simulink model "Bands6"  (R2018a)
settings: Solver=VariableStepAuto  StartTime=0.0  StopTime=0.01  RelTol=1e-3
undefined symbols (not defined in the file): fdesignblkfcn, G1, G2, G3, G4, G5, G6, gcbh, get, T
libraries: dspsrcs4 x1, dspxfrm3 x1, dspobslib x1
(part 1 of 2)
settings Model: Creator=Daniel  LastModifiedBy=Daniel

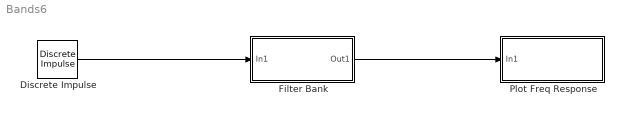
== system Bands6 ==
  Discrete Impulse : dspsrcs4/Discrete  Impulse  Delay=0  SampleTime=T  FrameSample=128  OutputFrames=off  dataType=double  isSigned=on  wordLen=16  udDataType=sfix(16)  fracBitsMode=Best precision  numFracBits=15  OutDataTypeStr=double  LastOutDataTypeStr=double
  "Filter Bank " : Subsystem
  Plot Freq Response : Subsystem
  wires:
  Discrete Impulse/1 -> "Filter Bank "/1(In1)
  "Filter Bank "/1(Out1) -> Plot Freq Response/1(In1)

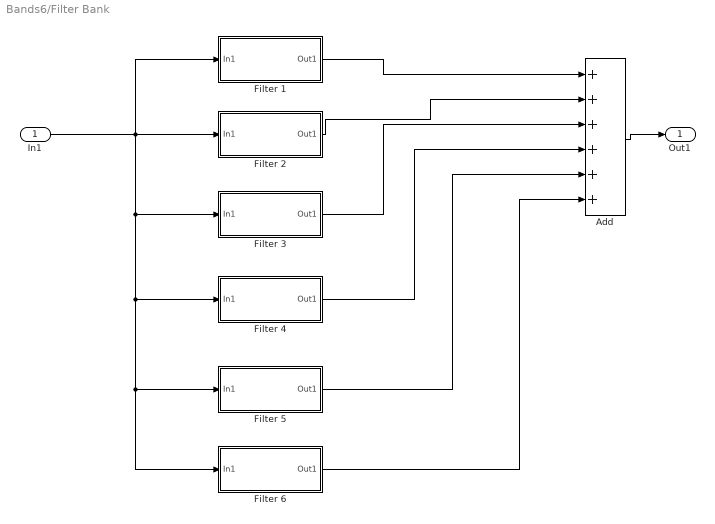
== system Bands6/Filter Bank  ==
  In1 : Inport
  Add : Sum  Inputs=++++++
  Filter 1 : Subsystem
  Filter 2 : Subsystem
  Filter 3 : Subsystem
  Filter 4 : Subsystem
  Filter 5 : Subsystem
  Filter 6 : Subsystem
  Out1 : Outport
  wires:
  In1/1 -> Filter 3/1(In1), Filter 6/1(In1), Filter 5/1(In1), Filter 4/1(In1), Filter 1/1(In1), Filter 2/1(In1)
  Add/1 -> Out1/1
  Filter 1/1(Out1) -> Add/1
  Filter 2/1(Out1) -> Add/2
  Filter 3/1(Out1) -> Add/3
  Filter 4/1(Out1) -> Add/4
  Filter 5/1(Out1) -> Add/5
  Filter 6/1(Out1) -> Add/6

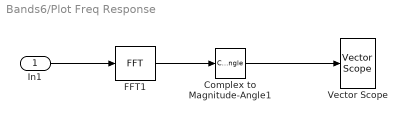
== system Bands6/Plot Freq Response ==
  In1 : Inport
  Complex to Magnitude-Angle1 : ComplexToMagnitudeAngle  Output=Magnitude
  FFT1 : dspxfrm3/FFT  FFTImplementation=Auto  CompMethod=Table lookup  TableOpt=NEW  TableOptActive=Speed  BitRevOrder=off  Normalize=off  InheritFFTLength=on  FFTLength=64  WrapInput=on  roundingMode=Floor  overflowMode=off  firstCoeffDataTypeStr=Inherit: Same word length as input  firstCoeffLastDataTypeStr=Inherit: Same word length as input  outputMin=[]  outputMax=[]
  Vector Scope : dspobslib/Vector Scope  ScopeProperties=off  Domain=Frequency  HorizSpan=1  DisplayProperties=off  AxisGrid=on  Memory=off  FrameNumber=off  AxisLegend=off  AxisZoom=off  OpenScopeAtSimStart=on  OpenScopeImmediately=off  FigPos=get(0,'defaultfigureposition')  AxisProperties=on  XUnits=Hertz  XRange=[0...Fs/2]  InheritXIncr=on  XIncr=1  XLabel=Samples  XLimit=Auto  XMin=0  XMax=1  XStart=0  YUnits=dB  YLabel=|Magnitude (dB)|  LineProperties=off  XAxisParamsVer=6.9
      settings: SourceProductName=DSP System Toolbox  SourceProductBaseCode=DS  YMin=0.0723692553519949  YMax=69.3188381671759
  wires:
  In1/1 -> FFT1/1
  FFT1/1 -> Complex to Magnitude-Angle1/1
  Complex to Magnitude-Angle1/1 -> Vector Scope/1

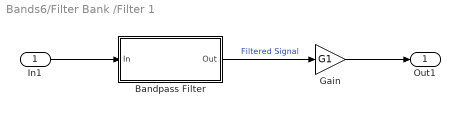
== system Bands6/Filter Bank /Filter 1 ==
  In1 : Inport
  Bandpass Filter : Subsystem  DialogController=fdesignblkfcn  InitFcn=fdesignblkfcn(gcbh, {'InitFcn'});  mask(Bandpass Filter){}
      mask help: Design a bandpass filter
      settings: CopyFcn=fdesignblkfcn(gcbh, {'CopyFcn'});
      mask Help: helpview(mapfilelocation('dsp'), 'dspbandpassfilter');
      mask Display: disp('Bandpass');
  Gain : Gain  Gain=G1
  Out1 : Outport
  wires:
  Bandpass Filter/1(Out) -> Gain/1  "Filtered Signal"
  In1/1 -> Bandpass Filter/1(In)
  Gain/1 -> Out1/1

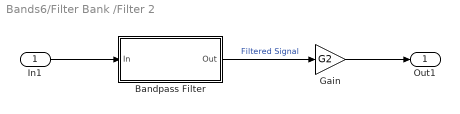
== system Bands6/Filter Bank /Filter 2 ==
  In1 : Inport
  Bandpass Filter : Subsystem  DialogController=fdesignblkfcn  InitFcn=fdesignblkfcn(gcbh, {'InitFcn'});  mask(Bandpass Filter){}
      mask help: Design a bandpass filter
      settings: CopyFcn=fdesignblkfcn(gcbh, {'CopyFcn'});
      mask Help: helpview(mapfilelocation('dsp'), 'dspbandpassfilter');
      mask Display: disp('Bandpass');
  Gain : Gain  Gain=G2
  Out1 : Outport
  wires:
  Bandpass Filter/1(Out) -> Gain/1  "Filtered Signal"
  In1/1 -> Bandpass Filter/1(In)
  Gain/1 -> Out1/1

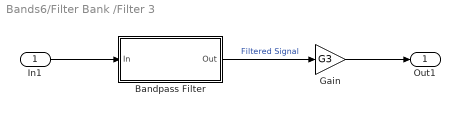
== system Bands6/Filter Bank /Filter 3 ==
  In1 : Inport
  Bandpass Filter : Subsystem  DialogController=fdesignblkfcn  InitFcn=fdesignblkfcn(gcbh, {'InitFcn'});  mask(Bandpass Filter){}
      mask help: Design a bandpass filter
      settings: CopyFcn=fdesignblkfcn(gcbh, {'CopyFcn'});
      mask Help: helpview(mapfilelocation('dsp'), 'dspbandpassfilter');
      mask Display: disp('Bandpass');
  Gain : Gain  Gain=G3
  Out1 : Outport
  wires:
  Bandpass Filter/1(Out) -> Gain/1  "Filtered Signal"
  In1/1 -> Bandpass Filter/1(In)
  Gain/1 -> Out1/1

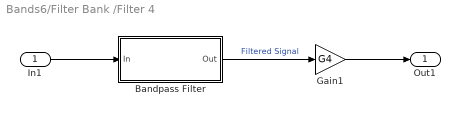
== system Bands6/Filter Bank /Filter 4 ==
  In1 : Inport
  Bandpass Filter : Subsystem  DialogController=fdesignblkfcn  InitFcn=fdesignblkfcn(gcbh, {'InitFcn'});  mask(Bandpass Filter){}
      mask help: Design a bandpass filter
      settings: CopyFcn=fdesignblkfcn(gcbh, {'CopyFcn'});
      mask Help: helpview(mapfilelocation('dsp'), 'dspbandpassfilter');
      mask Display: disp('Bandpass');
  Gain1 : Gain  Gain=G4
  Out1 : Outport
  wires:
  Bandpass Filter/1(Out) -> Gain1/1  "Filtered Signal"
  In1/1 -> Bandpass Filter/1(In)
  Gain1/1 -> Out1/1

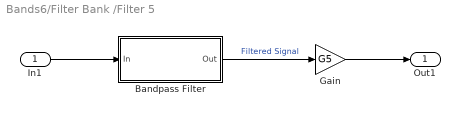
== system Bands6/Filter Bank /Filter 5 ==
  In1 : Inport
  Bandpass Filter : Subsystem  DialogController=fdesignblkfcn  InitFcn=fdesignblkfcn(gcbh, {'InitFcn'});  mask(Bandpass Filter){}
      mask help: Design a bandpass filter
      settings: CopyFcn=fdesignblkfcn(gcbh, {'CopyFcn'});
      mask Help: helpview(mapfilelocation('dsp'), 'dspbandpassfilter');
      mask Display: disp('Bandpass');
  Gain : Gain  Gain=G5
  Out1 : Outport
  wires:
  Bandpass Filter/1(Out) -> Gain/1  "Filtered Signal"
  In1/1 -> Bandpass Filter/1(In)
  Gain/1 -> Out1/1

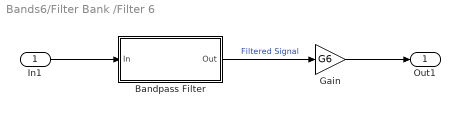
== system Bands6/Filter Bank /Filter 6 ==
  In1 : Inport
  Bandpass Filter : Subsystem  DialogController=fdesignblkfcn  InitFcn=fdesignblkfcn(gcbh, {'InitFcn'});  mask(Bandpass Filter){}
      mask help: Design a bandpass filter
      settings: CopyFcn=fdesignblkfcn(gcbh, {'CopyFcn'});
      mask Help: helpview(mapfilelocation('dsp'), 'dspbandpassfilter');
      mask Display: disp('Bandpass');
  Gain : Gain  Gain=G6
  Out1 : Outport
  wires:
  Bandpass Filter/1(Out) -> Gain/1  "Filtered Signal"
  In1/1 -> Bandpass Filter/1(In)
  Gain/1 -> Out1/1

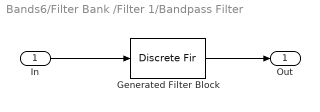
== system Bands6/Filter Bank /Filter 1/Bandpass Filter ==
  In : Inport
  Generated Filter Block : DiscreteFir  Tag=BlockMethodSubSystem  Coefficients=[-7.03055845481479099e-06 -2.29085807188983683e-05 -5.7003547719814073e-05 -0.000119567762253850577 -0.000222949707930134825 -0.000379897999978592198 -0.000601341554597424762 -0.00089353958713466494 -0.00125503282289146797 -0.00167391293164171804 -0.00212608340261492227 -0.00257516315481537417 -0.00297453765048486798 -0.00327173425265281717 -0.00341491553990109662 -0.00336079256760920186 -0.00308282116694620157 -0.00257825777237225256 -0.00187259228944337461 -0.00102007769837810978 -9.95993988954529301e-05 0.000794108626292330897 0.00156302489086289462 0.00212046622511692911 0.00240543193630230216 0.00239406806810692424 0.002105888060837619 0.00160310087723703897 0.000982525164113468193 0.000360922255027195228 -0.000144082905566220095 -0.000434290951166614592 -0.000448724115510219345 -0.000175427844251711563 0.000345315434149779017 0.00102744786704335152 0.0017545235230948834 0.00240144395679171667 0.00285855222687966424 0.00305339795404349894 0.00296571262293447973 0.00263229026298860119 0.00214039353017191286 0.0016106141889437786 0.0011723635394834727 0.000936851353408847155 0.00097315807450574208 0.00129258045330523947 0.00184488400813699865 0.00252767797097565349 0.00320734484102967949 0.00374737797037305153 0.00403820251928643011 0.00402198593914121147 0.00370679490786867457 0.00316658260313637139 0.002526502415741995 0.00193629019751401796 0.00153724329270419182 0.00142997675630323023 0.0016502559173649043 0.00215867071599457061 0.00284702345698311992 0.0035606171281857466 0.0041319845531319413 0.00441879925011210047 0.00433745931722841118 0.00388446812178028754 0.00314021368417176242 0.00225356255713334442 0.00141004292008724405 0.000790289414888854617 0.000527961065431415246 0.000676851673978991772 0.00119520535476166857 0.00195159669902519916 0.00275192069880885858 0.00338210444701678679 0.00365726674610375273 0.00346613902300582123 0.00280018315833446179 0.00175994389212322613 0.000536168970401300934 -0.000630987068028085398 -0.00150608059292994595 -0.0019137317022492671 -0.00178229362569573102 -0.0011650891378250294 -0.000233238394039379771 0.000759493511314397914 0.0015328213054930219 0.00184478260110618815 0.00155045175911886022 0.000640441596718928125 -0.000750768191946483195 -0.00236999934724997467 -0.00389962769947598507 -0.00502946858066383347 -0.00553016346579587783 -0.00531085129227605677 -0.00444681235614551897 -0.00316919412566554672 -0.00181749170706887336 -0.000764270530626963321 -0.00032859509084681238 -0.000698062914688417509 -0.00187823672611164968 -0.00368269561041871443 -0.00576796401947804373 -0.00770720214647630398 -0.0090871030058391547 -0.00960623462186278691 -0.00915167753168281105 -0.00783482068425727339 -0.00597587986548174088 -0.0040382952501647534 -0.0025260328740815104 -0.0018662072048435598 -0.00230400268267090622 -0.00383531966866586206 -0.00619494369166633321 -0.00890585619980482218 -0.0113811788586910961 -0.0130574188640829869 -0.0135292078346802847 -0.012653834955581169 -0.0105993165115266085 -0.0078216451775402953 -0.00497274098004035336 -0.00275699899069870719 -0.0017673679844909427 -0.00233840532416865069 -0.00445184358358078139 -0.00771989742636700234 -0.0114547570869246752 -0.0148130371381259129 -0.0169857627567569398 -0.0173921101918181505 -0.0158317356259817001 -0.0125574419433930624 -0.00824610674982560396 -0.0038680573755789753 -0.000478634564092539415 0.00102476596777190143 0.000126084011447518139 -0.00315876904003738407 -0.00824408482637618498 -0.0140663118243368659 -0.0192942977789984753 -0.0226186083714105327 -0.0230599590487757938 -0.0202281037416631934 -0.0144685309582597947 -0.00685462322192184267 0.000986081016009743858 0.00718732133241212386 0.0100443781066538607 0.00841971881574130401 0.00206753805888403464 -0.00819846555334263413 -0.0205423096399800671 -0.0323570754484899664 -0.0406962580552230058 -0.0428123672452970297 -0.0367041465511276088 -0.0215665024738620273 0.00194923977872560827 0.0317247384745718147 0.0644282771362778145 0.0959974281621706615 ...(+4093 chars)]  InputProcessing=Columns as channels (frame based)
  Out : Outport
  wires:
  In/1 -> Generated Filter Block/1
  Generated Filter Block/1 -> Out/1

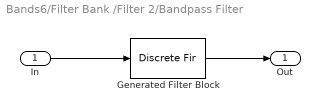
== system Bands6/Filter Bank /Filter 2/Bandpass Filter ==
  In : Inport
  Generated Filter Block : DiscreteFir  Tag=BlockMethodSubSystem  Coefficients=[1.42890450429576339e-06 6.04999333597359974e-06 1.46172851875464679e-05 2.33807022625062644e-05 2.19978787194749639e-05 -3.09489245658148342e-06 -5.78508557098895401e-05 -0.000126169147088056285 -0.000163553058094270535 -0.000111642666667859683 6.30831487681068209e-05 0.000323434964748066259 0.000542457995596972798 0.000543758771726919111 0.000202869782904821104 -0.000436188163665018772 -0.00110982592208898811 -0.00141630780882092419 -0.00102666418974686822 7.40938399023693441e-05 0.00147149497999503678 0.00245116920147764664 0.00235830500085235095 0.00101080585167346161 -0.0010906528941221523 -0.00293393995048066509 -0.0035100945393835405 -0.00240070692058710899 -7.8709437310937728e-05 0.00229863999761510977 0.0035214088089780683 0.00301843003801455885 0.00117867445254615831 -0.000909362176875266751 -0.00213991528729664832 -0.00205215533142274597 -0.00104143800857203479 4.75013759459243798e-06 0.000373071756239738575 1.31534580226656806e-05 -0.000495103817613226681 -0.000453480415519837642 0.000360882499460775667 0.00147826321474135323 0.00206840565296789692 0.00157474048828060327 0.000166120359684418279 -0.00134692212999075467 -0.00207881811727289416 -0.00169386808013713766 -0.000616548919935115138 0.000328241557594468377 0.000559134526182369462 0.00016108905493924795 -0.000241141041480270716 -4.81422975987580426e-05 0.000773872008639377401 0.00162433810461145461 0.00173845550791712771 0.000823108591910013429 -0.000659879594808484519 -0.00180654729362361407 -0.00194351632054725926 -0.00112695056238564092 -6.67348761690625565e-05 0.000462830932628293073 0.000244741475544102557 -0.00023750086509377461 -0.000254258718369672224 0.000497344144412273956 0.001572442344121868 0.00209778025500272341 0.0014869473896730245 -3.62811125522573773e-05 -0.00155502489067329023 -0.00214473372566695818 -0.00157891911551675764 -0.000475800464701522561 0.000240142610420348863 0.000117711793407833436 -0.000454968278963447433 -0.000614997061099885399 0.000178398769661815558 0.0015931581958745669 0.0026120057620096929 0.00233709392591583852 0.000756244779300734938 -0.00118106653527215878 -0.00227229538903139447 -0.00199081670287733908 -0.000868306799775584739 -3.73984899742101681e-06 -0.000103413586625566016 -0.000864931772854024257 -0.00124511213753075679 -0.000406633450307746056 0.00145721199116601616 0.00315022494150633695 0.00338186342391299903 0.00182831394962424776 -0.000547643134955088772 -0.00221958490116577322 -0.00229233816963695346 -0.00117965642444097072 -0.000186428571606007926 -0.00033525788556003957 -0.00143474180603354981 -0.00220935826013390034 -0.0014201966884710164 0.000959626439539171651 0.0035439317889976521 0.00454431651034929024 0.00319774323262079184 0.000420443990784640366 -0.00189438757752275334 -0.00238667853768951069 -0.00129460700021095162 -0.000164581020899594679 -0.000431135060357891399 -0.00207320269361803162 -0.00352995777197677614 -0.00301118528975759161 -0.000127217007976307547 0.00357027727952318168 0.005675960735351291 0.00481099328870686696 0.00174082097803146237 -0.0012395773722729687 -0.00218341192928595126 -0.00107079264663875284 0.000265092475503371191 -0.000162873995554960584 -0.00260797830497225399 -0.00517196173859410177 -0.00530871099099323486 -0.00204590161311201356 0.0029692269025839769 0.00657889202860406121 0.00655326256053943932 0.0033554355954590635 -0.00027900439085199835 -0.00164997926547989738 -0.000364864191815439626 0.00138247524738430941 0.000827191954886914022 -0.00274022016259495684 -0.00703263238633063115 -0.0084510452036771315 -0.00509553420904184165 0.00142678171130683484 0.00702955518327943226 0.00829176713903050783 0.00515168199228403616 0.00085660367430645968 -0.000866005409048060709 0.000937513091840247383 0.00358172044115443681 0.0031227033067627607 -0.00195439987718252356 -0.00893317226717498317 -0.0126833214426922188 -0.00978138184748714341 -0.00153216184975563802 0.00677323060312540713 0.00994508690983661459 0.0070188905117505411 0.00191111947500218729 -7.89669679776224573e-05 ...(+5675 chars)]  InputProcessing=Columns as channels (frame based)
  Out : Outport
  wires:
  In/1 -> Generated Filter Block/1
  Generated Filter Block/1 -> Out/1

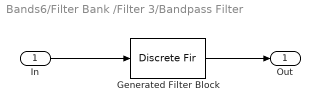
== system Bands6/Filter Bank /Filter 3/Bandpass Filter ==
  In : Inport
  Generated Filter Block : DiscreteFir  Tag=BlockMethodSubSystem  Coefficients=[-4.020149035064062e-07 -9.72078154206768929e-07 1.63565130366598736e-07 4.04386068899547807e-06 5.48921321832161013e-06 -4.02925832111594654e-06 -1.94973855299333424e-05 -1.44506698194799961e-05 2.66152747606277309e-05 6.13137556897496821e-05 1.49977699545525338e-05 -0.000101594420644433107 -0.000135806589409686104 3.89746355022413626e-05 0.000272640389536664147 0.00020866194504297225 -0.000232908281814967833 -0.000551610841164454943 -0.000172543915606090503 0.0006535083034006294 0.000854083143981365514 -0.000138312548067845176 -0.00129627772408214795 -0.000967275825315495712 0.000847552445933638979 0.00197074929737175476 0.000625289028826512693 -0.00187916452618936314 -0.00231007698232046747 0.000293923021730961294 0.00286738737037543334 0.00196136187614633431 -0.00156443012921809663 -0.00327896478912245324 -0.000886714815566765849 0.00260547049251120709 0.00275886306409840916 -0.000459583422453290836 -0.00279088314935687851 -0.00148063063385879415 0.00131316656671037215 0.00192830089535178488 0.00016784508892643546 -0.00112082219855159601 -0.000521966270701166028 0.000358241441102661803 3.06247792683182125e-05 -0.000500829049782927508 0.000170524287228238314 0.00111915447696509939 0.000493089331756113515 -0.00118023796560301291 -0.0014268306372631572 0.000342371021968022676 0.00168110509836347298 0.000702198991089900484 -0.00108560069777294071 -0.00113149669734124753 0.00032933378306140436 0.000919021044223735685 -3.28266020823822285e-05 -0.000674473196682178443 7.90355313254347447e-05 0.000771947927093317521 3.15490635292707509e-05 -0.000966764840624439038 -0.000444590681208169704 0.000879403934472279352 0.000853614413264367432 -0.000525923286828168177 -0.00102188774475288628 0.000168646415546735176 0.00105310750330673262 0.000136803116954048589 -0.0010658908988878525 -0.000525039252261902162 0.000916733031998552984 0.000919014496901856799 -0.000492656989377563228 -0.00101769730362383259 6.84695368230828645e-05 0.00080659714980303276 6.89801048736893822e-07 -0.00073854792909894035 9.81797051579360946e-05 0.0010963531721019772 0.000242488619733197309 -0.00140193263784559041 -0.00112658273393288983 0.000937531230344820494 0.00175917560208187088 0.000144610426784509168 -0.00141287898590732627 -0.000787257813273429695 0.000564249335388721852 0.000416582469710923128 -0.000426012199346413264 9.79654030385104313e-05 0.00123520210727289859 0.000489785404151604612 -0.00169246935755029866 -0.00193909810139086358 0.000650560172982174922 0.00256967571832459035 0.00110490912477632583 -0.00150079989487324249 -0.00167192749823861955 7.09714954717263324e-05 0.000647588506782316138 -0.000169099679784318654 0.000103942711618108951 0.00151109153302971737 0.0010471762710927287 -0.00178319125456461456 -0.00300309899517426987 -0.000165453488820727985 0.00317375874052859379 0.00243155872579596749 -0.0010906837711844215 -0.00244568317704509618 -0.000667166784476881094 0.000621835511516282075 -7.3143281743777845e-05 -1.37585548975354282e-05 0.00185723247713436988 0.00204050029886806853 -0.0014062925093718294 -0.00417991589236894109 -0.00168332175874285933 0.00325421527405025772 0.00399225205015207342 -3.18130717573725e-05 -0.00286982128051678845 -0.0015205129493653935 0.000335480729706896124 -0.000246265248199245622 -0.000464086641292408664 0.00207272329492002054 0.00350722608574966779 -0.000227323830762122701 -0.0051428312329060092 -0.00394491115779141335 0.00243754677538245666 0.0054734179867220404 0.00168933107307944102 -0.00270146420016404744 -0.00224033837274485422 -6.49197021553388562e-05 -0.000707766206599564469 -0.0015074278992936467 0.00177317654911073258 0.00531397152585509538 0.00209960032753673349 -0.00536864425243860615 -0.00679516483786562694 0.000373999827554664628 0.00641589339017230916 0.00390437521947194742 -0.001793906464500915 -0.00253169976650997539 -0.000255467590411307028 -0.00128033726032274545 -0.00336814630909219349 0.000379909151859683409 0.00707063106252888221 0.00585292524504125566 -0.00415939956327509002 ...(+6594 chars)]  InputProcessing=Columns as channels (frame based)
  Out : Outport
  wires:
  In/1 -> Generated Filter Block/1
  Generated Filter Block/1 -> Out/1

== system Bands6/Filter Bank /Filter 4/Bandpass Filter ==
  In : Inport
  Generated Filter Block : DiscreteFir  Tag=BlockMethodSubSystem  Coefficients=[4.91852730579905137e-08 -1.38944823607508147e-07 -2.79447440242863678e-07 6.74204198366025194e-07 7.44960528538658458e-07 -2.29914372088471355e-06 -1.29566480170485301e-06 6.21321821020350968e-06 1.08536566640830798e-06 -1.41530834986718946e-05 2.08726587220568902e-06 2.80220163401512478e-05 -1.25623572968690214e-05 -4.89554347422096607e-05 3.74078456519123968e-05 7.57223420887405993e-05 -8.63520329902647788e-05 -0.000102625710658662127 0.00017054168060595871 0.000117428212010770662 -0.000299766167877527393 -0.000100195170862613905 0.000478216579634998206 2.41415595049918009e-05 -0.000699508186479139908 0.000140591783694012269 0.000942414710239560991 -0.000419948485358855766 -0.0011692616540012273 0.000826554200647576748 0.00132888137645308384 -0.00134998621567262436 -0.00136521247641650106 0.00194984674635219801 0.00123103160953994895 -0.00255505756370012597 -0.000904256652260455591 0.00307191176996093494 0.000402393655485099055 -0.00340127683476169418 0.000210197850943314124 0.00346233290130529541 -0.000826799634241165795 -0.00321720995408090538 0.00131653654989845651 0.00268899393760207907 -0.00155413710398723476 -0.00196583673483198161 0.00145465822268828291 0.00118681726988060393 -0.00100333402004703894 -0.000510359798869556604 0.000270157588514759856 7.20622819544113318e-05 0.000598217189984981369 5.63003411187231796e-05 -0.00141047264719198237 0.000106899794191113069 0.00197992896506828412 -0.000452264789821611073 -0.00217766536667503849 0.000807679973692584843 0.00197269488584932498 -0.000990026391986503773 -0.00144458165826186788 0.000865574205161853683 0.000761569344878384449 -0.000399379366340262812 -0.000128507798618711318 -0.000324525688875897014 -0.000280023122092556726 0.00112208241103044139 0.000379143467239672542 -0.00176431009981109521 -0.000203943380735451788 0.00205224224302431391 -0.000102475504215479086 -0.00188659998092547809 0.000341808184081101197 0.00130675120839296465 -0.000337414359426517919 -0.000482649421130155196 7.89068303189243271e-06 -0.000340381094643541653 0.000591128673265660029 0.000926445441895325694 -0.00127566829418122168 -0.00113336970343683326 0.00179340410334584551 0.000964423980823476967 -0.00191586705633639315 -0.000565776974231445664 0.00152957367581218855 0.000167712646317633971 -0.000690443844884983809 1.02512324924120044e-05 -0.000382610357070522643 0.000145662051262368064 0.00137697763038955212 -0.00058711738997675809 -0.00199587308646120192 0.00111187521649395017 0.00206781153697878535 -0.00143822651675247558 -0.00161289634663733575 0.00132027854275524334 0.00083712724929730514 -0.000659800414015033619 -5.30311200823927676e-05 -0.000432004217666670488 -0.000445252127486574288 0.00165280688563915852 0.000503767138456138607 -0.00260718586793347524 -0.000176746813484733085 0.00295126179937209559 -0.000291029119513399009 -0.0025290084183138932 0.000565838117737562795 0.00144438081620952086 -0.000373438725259581962 -3.54566891231545168e-05 -0.000365549971541364129 -0.00124547227723620195 0.00147258904019176512 0.00200293532282943545 -0.0025541671585186292 -0.00205344211528450974 0.0031425151321670705 0.00149982627119380038 -0.00288384512775573037 -0.000689209860017078908 0.00169945230649856433 6.55103280441210299e-05 0.000150083895632041587 2.72348093253113519e-05 -0.00213277444748550355 0.000490539529370372638 0.00362817901096868954 -0.00137512193061272575 -0.00415921553861396242 0.00214070320480027471 0.00358122083312741729 -0.00225744813945250207 -0.00214773280280712532 0.00139118473670603511 0.000418171065607932124 0.000415066588824675989 0.000963642516824082676 -0.00270161692190798181 -0.0015348831264702825 0.00472568459501825251 0.00121335566823480012 -0.00572845861924581052 -0.000341906581109584825 0.00523626845191283059 -0.0004520246586555828 -0.00327359648556056282 0.00053424932422170546 0.000392416113185960311 0.000431374283373686922 0.00250855184349832753 -0.0022825358315886092 -0.00451535502225569856 0.004360273705820099 0.00505430407704123789 -0.00573257610881400433 ...(+7178 chars)]  InputProcessing=Columns as channels (frame based)
  Out : Outport
  wires:
  In/1 -> Generated Filter Block/1
  Generated Filter Block/1 -> Out/1
